simulink model "MotorTest"  (R2015a)
settings: Solver=ode3  StartTime=0.0  StopTime=10.0  RelTol=1e-3
libraries: PoliArd x7, simulink x1
settings Model: ExtModeTrigDuration=2  Creator=User  LastModifiedBy=User
settings OptimizationCC: OptimizeModelRefInitCode=on  LifeSpan=1
settings DebuggingCC: UnderspecifiedInitializationDetection=Classic  MergeDetectMultiDrivingBlocksExec=none
settings HardwareCC: ProdLargestAtomicInteger=Long  ProdLargestAtomicFloat=Double  ProdEndianess=LittleEndian  ProdHWDeviceType=ARM Compatible->ARM Cortex
settings RTWCC: SystemTargetFile=realtime.tlc  GenerateMakefile=off  TemplateMakefile=realtime.tmf  Description=Run on Target Hardware  RTWVerbose=off
settings ERTTargetCC: CombineOutputUpdateFcns=off  ExtModeTransport=3  ExtModeMexFile=ext_serial_win32_comm_rtt  ExtModeMexArgs=0 1 9600  ERTSrcFileBannerTemplate=realtime_code_template.cgt  ERTHdrFileBannerTemplate=realtime_code_template.cgt  ERTDataSrcFileTemplate=realtime_code_template.cgt  ERTDataHdrFileTemplate=realtime_code_template.cgt  ERTCustomFileTemplate=realtime_file_process.tlc

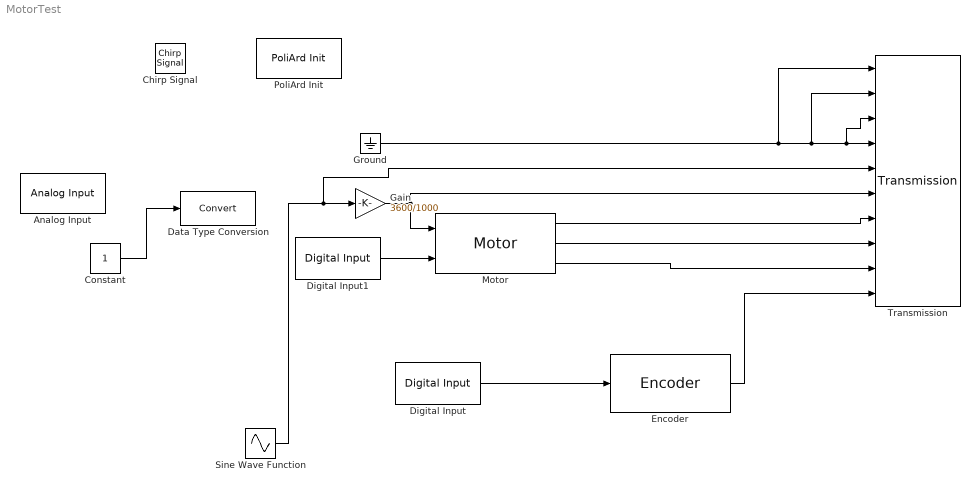
== system MotorTest ==
  Analog Input : PoliArd/Analog Input  AIpin_mask=8  AIsample=-1
  Chirp Signal : simulink/Sources/Chirp Signal  f1=5  T=30  f2=15
  Constant : Constant
  Data Type Conversion : DataTypeConversion
  Digital Input : PoliArd/Digital Input  DI_pin=2  DIsample=-1
  Digital Input1 : PoliArd/Digital Input  DI_pin=3  DIsample=-1
  Encoder : PoliArd/Encoder  EncoderID=1  dt_enc=-1
  Gain : Gain  Gain=3600/1000
  Ground : Ground
  Motor : PoliArd/Motor  MotorID=1  DC_bus_mask=12  dt_mot=-1
  PoliArd Init : PoliArd/PoliArd Init
  Sine Wave Function : Sin  Frequency=2*3.14  SampleTime=0
  Transmission : PoliArd/Transmission  sample_freq=100  sig_to_send=6
  wires:
  Encoder/1 -> Transmission/10
  Digital Input/1 -> Encoder/1
  Digital Input1/1 -> Motor/2
  Ground/1 -> Transmission/1, Transmission/2, Transmission/3, Transmission/4
  Motor/3 -> Transmission/9
  Motor/2 -> Transmission/8
  Motor/1 -> Transmission/7
  Gain/1 -> Transmission/6, Motor/1
  Constant/1 -> Data Type Conversion/1
  Sine Wave Function/1 -> Transmission/5, Gain/1
